simulink model "ReactionWheel0"  (R2018b)
settings: Solver=FixedStepAuto  StartTime=0.0  StopTime=50  FixedStep=0.025  RelTol=1e-3
InitFcn:
  | loadThrusterData
settings Model: Creator=Andy  LastModifiedBy=barthal
settings DataIOCC: SaveOutput=off  SaveTime=off
settings ModelReferenceCC: ModelReferenceNumInstancesAllowed=Single
settings RTWCC: GenCodeOnly=on

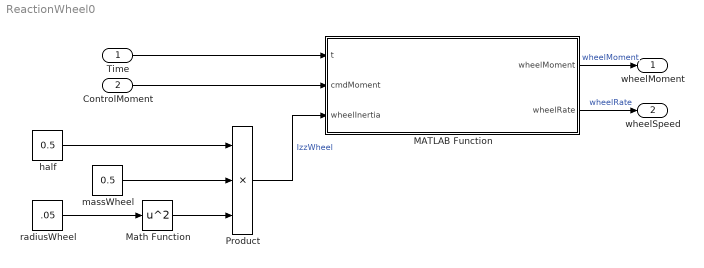
== system ReactionWheel0 ==
  Time : Inport  OutDataTypeStr=double  PortDimensions=1
  ControlMoment : Inport  Port=2  OutDataTypeStr=double  PortDimensions=1
  MATLAB Function : MATLAB Function  TreatAsAtomicUnit=on
  Math Function : Math  Operator=square  SaturateOnIntegerOverflow=on
  Product : Product  Inputs=3
  half : Constant  Value=0.5
  massWheel : Constant  Value=0.5
  radiusWheel : Constant  Value=.05
  wheelMoment : Outport  OutDataTypeStr=double  PortDimensions=1
  wheelSpeed : Outport  Port=2  OutDataTypeStr=double  PortDimensions=1
  wires:
  radiusWheel/1 -> Math Function/1
  Math Function/1 -> Product/3
  massWheel/1 -> Product/2
  half/1 -> Product/1
  Product/1 -> MATLAB Function/3(wheelInertia)  "IzzWheel"
  ControlMoment/1 -> MATLAB Function/2(cmdMoment)
  MATLAB Function/1(wheelMoment) -> wheelMoment/1  "wheelMoment"
  MATLAB Function/2(wheelRate) -> wheelSpeed/1  "wheelRate"
  Time/1 -> MATLAB Function/1(t)

== matlab function ReactionWheel0/MATLAB Function ==
  settings: updateMethod=DISCRETE
  data: wheelMoment output; wheelRate output; t input; cmdMoment input; wheelInertia input
function [wheelMoment,wheelRate] = callreactionWheel(t,cmdMoment,wheelInertia)

[wheelMoment,wheelRate] = reactionWheel(t,cmdMoment,wheelInertia);
